simulink model "states_5_B_double_simu"  (R2014b)
settings: Solver=ode45  StartTime=0.0  StopTime=100  RelTol=1e-3
values from neighbouring files (symbols this model uses):
  A = -1*[-1/L2 ... (first row only)    [ett_slap.m]    (also in linearss_circle.m = -1*[-1/L4 1/L3 0; states_5_linearss.m = -1*[0 1 0 0 0; tva_slap.m = -1*[-1/L3 1/L2)
  B = -1*[1/L1]'    [ett_slap.m]    (also in linearss_circle.m = -1*[0 0 1/L1]'; states_5_linearss.m = -1*[0 0 0 0 1/L1]'; tva_slap.m = -1*[0 1/L1]')
  C = eye(1)    [ett_slap.m]    (also in linearss_circle.m = eye(3); states_5_linearss.m = eye(5); tva_slap.m = eye(2))
  D = zeros(1,1)    [ett_slap.m]    (also in linearss_circle.m = zeros(3,1); states_5_linearss.m = zeros(5,1); tva_slap.m = zeros(2,1))
undefined symbols (not defined in the file or in its folder): K
libraries: simulink x2
settings Model: Creator=marcus  LastModifiedBy=marcus

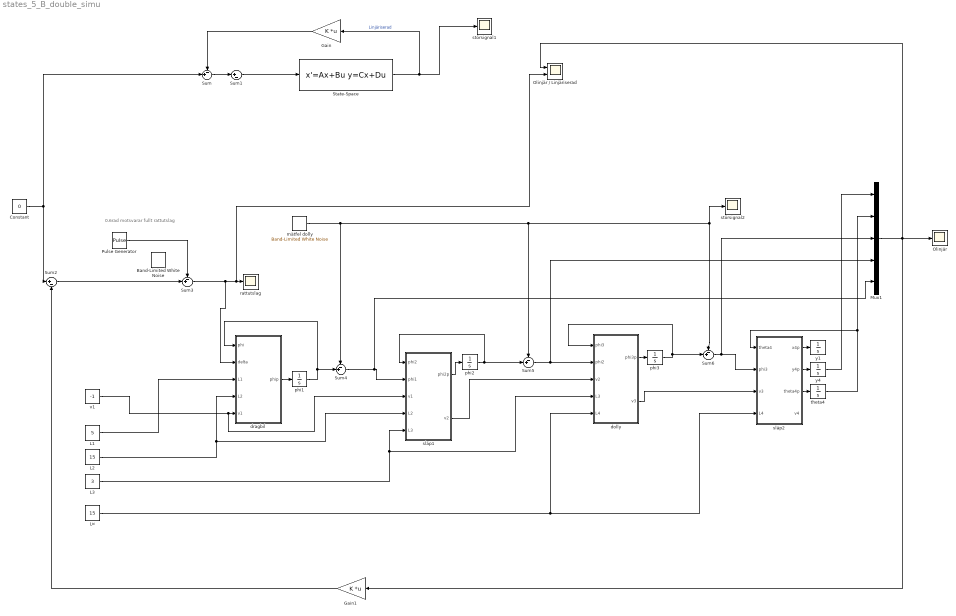
== system states_5_B_double_simu ==
  note: 0.6rad motsvarar fullt rattutslag
  Band-Limited White Noise : simulink/Sources/Band-Limited White Noise  Cov=[0.0001]  Ts=0.1  seed=[23341]
  Constant : Constant  Value=0
  Gain : Gain  Gain=K  Multiplication=Matrix(K*u)
  Gain1 : Gain  Gain=K  Multiplication=Matrix(K*u)
  L1 : Constant  Value=5  SampleTime=1
  L2 : Constant  Value=15  SampleTime=1
  L3 : Constant  Value=3  SampleTime=1
  L¤ : Constant  Value=15  SampleTime=1
  Mux1 : Mux  Inputs=5
  Olinjär : Scope
      settings: ShowLegends=on
  Olinjär / Linjäriserad : Scope  NumInputPorts=2
      settings: TickLabels=on  ShowLegends=on  YMin=-5~-5  YMax=5~5
  Pulse Generator : DiscretePulseGenerator  PulseType=Time based  Amplitude=0.0  Period=1000  PhaseDelay=5
  State-Space : StateSpace  A=A  B=B  C=C  D=D  X0=0
  Sum{,3..6} (5 alike) : Sum  Inputs=-+|
  Sum1 : Sum  Inputs=|+-
  Sum2 : Sum  Inputs=|+-
  dolly : MATLAB Function  TreatAsAtomicUnit=on
  dragbil : MATLAB Function  TreatAsAtomicUnit=on
  mätfel dolly : simulink/Sources/Band-Limited White Noise  Cov=[0.0000248]  Ts=0.1  seed=[23341]
  phi1 : Integrator
  phi2 : Integrator
  phi3 : Integrator
  rattutslag : Scope
      settings: ShowLegends=on  SaveName=ScopeData2
  släp1 : MATLAB Function  TreatAsAtomicUnit=on
  släp2 : MATLAB Function  TreatAsAtomicUnit=on
  störsignal1 : Scope
      settings: ShowLegends=on  SaveName=ScopeData4
  störsignal2 : Scope
      settings: ShowLegends=on  SaveName=ScopeData5
  theta4 : Integrator
  v1 : Constant  Value=-1  SampleTime=1
  y1 : Integrator
  y4 : Integrator
  wires:
  Constant/1 -> Sum/2, Sum2/1
  dolly/1(phi3p) -> phi3/1
  släp1/1(phi2p) -> phi2/1
  dragbil/1(phip) -> phi1/1
  släp2/3(theta4p) -> theta4/1
  släp2/2(y4p) -> y4/1
  v1/1 -> släp1/3(v1), dragbil/5(v1)
  L2/1 -> dragbil/4(L2), släp1/4(L2)
  L1/1 -> dragbil/3(L1)
  Sum1/1 -> State-Space/1
  dolly/2(v3) -> släp2/3(v3)
  släp1/2(v2) -> dolly/3(v2)
  y4/1 -> Mux1/1
  theta4/1 -> släp2/1(theta4), Mux1/2
  Mux1/1 -> Gain1/1, Olinjär / Linjäriserad/1, Olinjär/1
  L3/1 -> dolly/4(L3), släp1/5(L3)
  L¤/1 -> dolly/5(L4), släp2/4(L4)
  State-Space/1 -> Gain/1, störsignal1/1  "Linjäriserad"
  Sum2/1 -> Sum3/2
  Gain/1 -> Sum/1
  Sum/1 -> Sum1/1
  phi3/1 -> Sum6/2, dolly/1(phi3)
  mätfel dolly/1 -> Sum6/1, störsignal2/1, Sum5/1, Sum4/1
  phi2/1 -> Sum5/2, släp1/1(phi2)
  Sum5/1 -> Mux1/4, dolly/2(phi2)
  Sum6/1 -> Mux1/3, släp2/2(phi3)
  phi1/1 -> Sum4/2, dragbil/1(phi)
  Sum4/1 -> Mux1/5, släp1/2(phi1)
  Pulse Generator/1 -> Sum3/1
  Sum3/1 -> Olinjär / Linjäriserad/2, rattutslag/1, dragbil/2(delta)
  Gain1/1 -> Sum2/2
  släp2/1(x4p) -> y1/1

== matlab function states_5_B_double_simu/släp1 ==
  data: phi2 input; phi1 input; v1 input; phi2p output; L2 input; L3 input; v2 output
function [phi2p,v2]= fcn(phi2,phi1,v1,L2,L3)
%#codegen


v2 = v1*cos(phi1);
phi2p = v2*(tan(phi1)/L2-sin(phi2)/L3);

== matlab function states_5_B_double_simu/dragbil ==
  data: phi input; delta input; phip output; L1 input; L2 input; v1 input
function phip = fcn(phi,delta,L1,L2,v1)
%#codegen

phip = v1*(tan(delta)/L1-sin(phi)/L2);

== matlab function states_5_B_double_simu/dolly ==
  data: phi3 input; phi2 input; v2 input; L3 input; phi3p output; L4 input; v3 output
function [phi3p,v3]= fcn(phi3,phi2,v2,L3,L4)
%#codegen

v3 = v2*cos(phi2);
phi3p = v3*(tan(phi2)/L3-sin(phi3)/L4);

== matlab function states_5_B_double_simu/släp2 ==
  data: theta4 input; phi3 input; v3 input; x4p output; L4 input; y4p output; theta4p output; v4 output
function [x4p,y4p,theta4p,v4]= fcn(theta4,phi3,v3,L4)
%#codegen

v4 = v3*cos(phi3);
theta4p=v4*tan(phi3)/L4;
x4p=v4*cos(theta4);
y4p=v4*sin(theta4);
